simulink model "CompleteDronePathSimulation"  (R2022b)
settings: Solver=VariableStepAuto  StartTime=0.0  StopTime=10.0  RelTol=1e-3
settings Model: Creator=zs  LastModifiedBy=zs

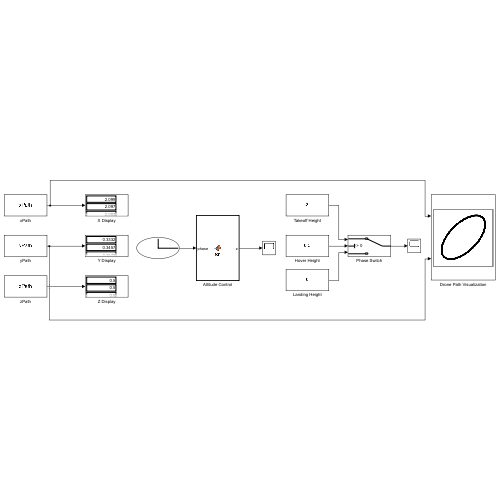
[thumbnail: Simulink's stored preview of the top-level diagram]
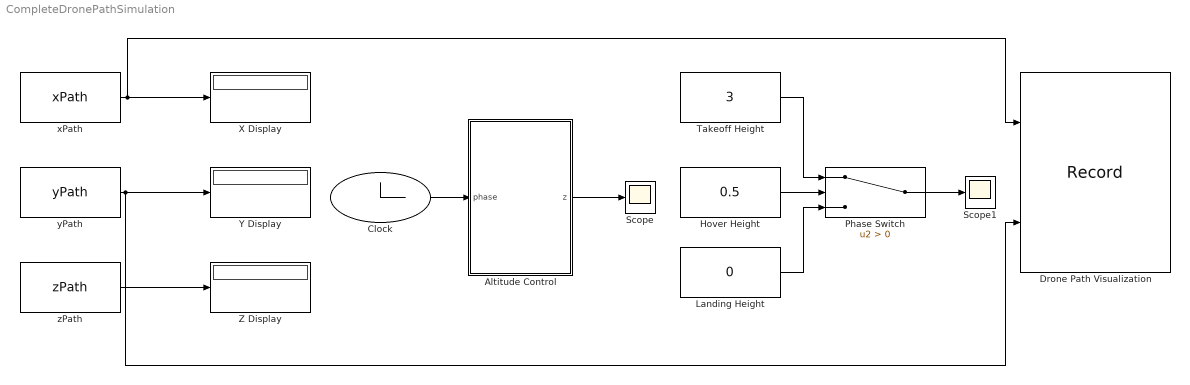
== system CompleteDronePathSimulation ==
  Altitude Control : MATLAB Function  TreatAsAtomicUnit=on
  Clock : Clock
  Drone Path Visualization : Record  FileSettingsInternal="{\"entries\":[{\"content\":{\"excelSettings\":{\"content\":{},\"type\":\"Streamout.ExcelSettings\"}},\"type\":\"Streamout.FileSettingStorage\",\"uuid\":\"8648b853-ad2b-493e-be67-094b35974909\"}],\"packageUris\":[\"http://schema.mathworks.com/mf0/streamout_blocks/R2020a\"],\"version\":\"1.0\"}"  Layout=[1 1]  SignalsInternal="{\"entries\":[{\"content\":{\"signals\":[{\"content\":{\"blockPath\":[\"CompleteDronePathSimulation/Drone Path Visualization\"],\"channel\":[],\"dimensions\":[179],\"domain\":\"CompleteDronePathSimulation/Drone Path Visualization\",\"hasChildren\":true,\"lineColor\":\"#64d413\",\"plots\":[],\"port\":1,\"sid\":[\"\"],\"signalID\":206,\"signalName\":\"xPath\"},\"type\":\"RecordBlkView.Signal\",\"uuid\":\"f33c3a68-aaaa-478f-b7c3-6c0a5d6fe465\"},{\"content\":{\"blockPath\":[\"CompleteDronePathSimulation/Drone Path Visualization\"],\"channel\":[1],\"dimensions\":[179],\"domain\":\"CompleteDronePathSimulation/Drone Path Visualization\",\"lineColor\":\"#ff13a6\",\"parentID\":206,\"plots\":[],\"port\":1,\"sid\":[\"\"],\"signalID\":207,\"signalName\":\"xPath\"},\"type\":\"RecordBlkView.Signal\",\"uuid\":\"267a787f-4a79-4fd0-86c7-f56c86156cb3\"},{\"content\":{\"blockPath\":[\"CompleteDronePathSimulation/Drone Path Visualization\"],\"channel\":[],\"dimensions\":[179],\"domain\":\"CompleteDronePathSimulation/Drone Path Visualization\",\"hasChildren\":true,\"lineColor\":\"#fe330a\",\"plots\":[],\"port\":2,\"sid\":[\"\"],\"signalID\":211,\"signalName\":\"yPath\"},\"type\":\"RecordBlkView.Signal\",\"uuid\":\"d36d66b1-ff61-46db-80cc-8c7404fc5444\"},{\"content\":{\"blockPath\":[\"CompleteDronePathSimulation/Drone Path Visualization\"],\"channel\":[1],\"dimensions\":[179],\"domain\":\"CompleteDronePathSimulation/Drone Path Visualization\",\"lineColor\":\"#22b573\",\"parentID\":211,\"plots\":[],\"port\":2,\"sid\":[\"\"],\"signalID\":212,\"signalName\":\"yPath\"},\"type\":\"RecordBlkView.Signal\",\"uuid\":\"76d9c800-666b-4678-ab27-f05f3a6e85f2\"}]},\"type\":\"RecordBlkView.InputSignals\",\"uuid\":\"50173eea-ada1-40e6-b297-6a62602d1254\"}],\"packageUris\":[\"http://schema.mathworks.com/mf0/streamout_blocks/R2020a\"],\"version\":\"1.0\"}"  VisualizationBindings="{\"xyplotplugin\":{\"info\":[{\"series\":[],\"subplotID\":1}]}}"  CompatibilityTag=XY
  Hover Height : Constant  Value=0.5
  Landing Height : Constant  Value=0
  Phase Switch : Switch  Criteria=u2 > Threshold  SaturateOnIntegerOverflow=off  InputSameDT=off
  Scope : Scope
  Scope1 : Scope
  Takeoff Height : Constant  Value=3
  X Display : Display
  Y Display : Display
  Z Display : Display
  xPath : FromWorkspace  VariableName=xPath
  yPath : FromWorkspace  VariableName=yPath
  zPath : FromWorkspace  VariableName=zPath
  wires:
  xPath/1 -> X Display/1, Drone Path Visualization/1
  yPath/1 -> Drone Path Visualization/2, Y Display/1
  zPath/1 -> Z Display/1
  Clock/1 -> Altitude Control/1(phase)
  Takeoff Height/1 -> Phase Switch/1
  Hover Height/1 -> Phase Switch/2
  Landing Height/1 -> Phase Switch/3
  Altitude Control/1(z) -> Scope/1
  Phase Switch/1 -> Scope1/1

== matlab function CompleteDronePathSimulation/Altitude Control ==
  data: phase input; z output
function z = fcn(phase)
    if phase == 1
        z = 3;       % Takeoff height
    elseif phase == 2
        z = 1.5;     % Hover height
    else
        z = 0;       % Landing height
    end
end
